simulink model "vtol50kg_hil_chuangheng"  (R2024b)
settings: Solver=FixedStepAuto  StartTime=0.0  StopTime=inf  FixedStep=5/1000  RelTol=1e-3
libraries: slrealtimeutilitieslib x42, slrealtimeiplib x3, simulink x2, aerolibatmos2 x1, hdlsllib x1
settings Model: DataDictionary=nextpilot_datadict.sldd  Creator=CETCA  LastModifiedBy=CETCA
settings DataIOCC: ExternalInput=getinputstruct(report8)  InitialState=getstatestruct(report8)

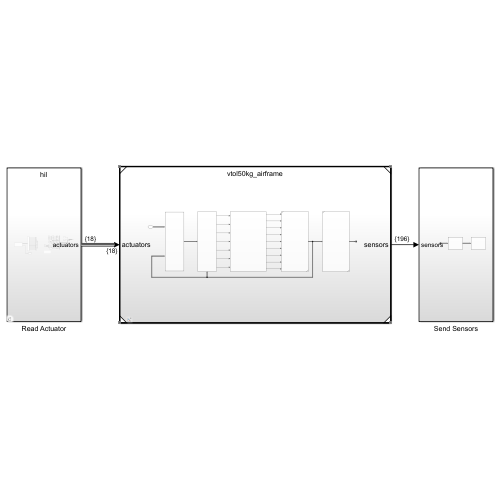
[thumbnail: Simulink's stored preview of the top-level diagram]
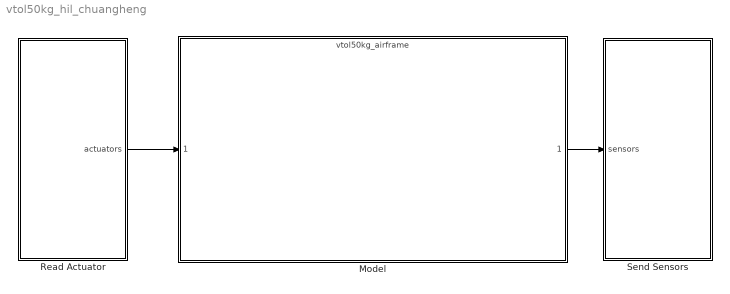
== system vtol50kg_hil_chuangheng ==
  Model : ModelReference  ModelNameDialog=vtol50kg_airframe.slx  SimulationMode=Normal  ModelReferenceVersion=5.134
  Read Actuator : Subsystem  Variant=on
  Send Sensors : Subsystem
  wires:
  Read Actuator/1(actuators) -> Model/1
  Model/1 -> Send Sensors/1(sensors)

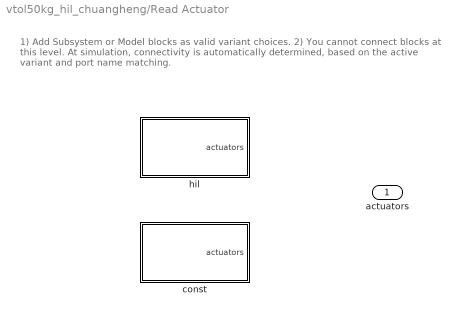
== system vtol50kg_hil_chuangheng/Read Actuator ==
  note: 1) Add Subsystem or Model blocks as valid variant choices.
      | 2) You cannot connect blocks at this level. At simulation, connectivity is automatically
      | determined, based on the active variant and port name matching.
  const : Subsystem  VariantControl=false
  hil : Subsystem  VariantControl=true
  actuators : Outport

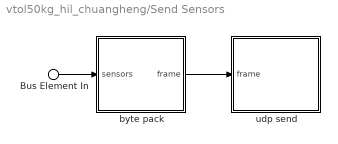
== system vtol50kg_hil_chuangheng/Send Sensors ==
  Bus Element In : Inport  PortName=sensors
  byte pack : Subsystem
  udp send : Subsystem
  wires:
  byte pack/1(frame) -> udp send/1(frame)
  Bus Element In/1 -> byte pack/1(sensors)

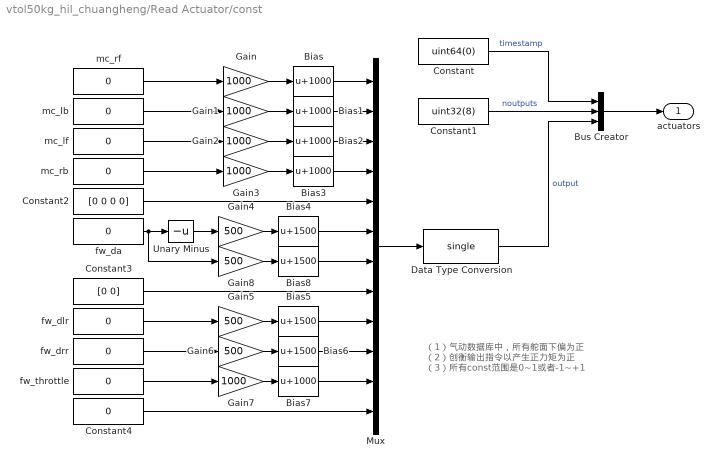
== system vtol50kg_hil_chuangheng/Read Actuator/const ==
  note: （1）气动数据库中，所有舵面下偏为正
      | （2）创衡输出指令以产生正力矩为正
      | （3）所有const范围是0~1或者-1~+1
  Bias{,1..3,7} (5 alike) : Bias  Bias=1000  SaturateOnIntegerOverflow=off
  Bias{4..6,8} (4 alike) : Bias  Bias=1500  SaturateOnIntegerOverflow=off
  Bus Creator : BusCreator  Inputs=3
  Constant : Constant  Value=uint64(0)
  Constant1 : Constant  Value=uint32(8)
  Constant2 : Constant  Value=[0 0 0 0]
  Constant3 : Constant  Value=[0 0]
  Constant4 : Constant  Value=0
  Data Type Conversion : DataTypeConversion  OutDataTypeStr=single  SaturateOnIntegerOverflow=off  RndMeth=Floor
  Gain{,1..3,7} (5 alike) : Gain  Gain=1000
  Gain{4..6,8} (4 alike) : Gain  Gain=500
  Mux : Mux  Inputs=12
  Unary Minus : UnaryMinus
  fw_da : Constant  Value=0
  fw_dlr : Constant  Value=0
  fw_drr : Constant  Value=0
  fw_throttle : Constant  Value=0
  mc_lb : Constant  Value=0
  mc_lf : Constant  Value=0
  mc_rb : Constant  Value=0
  mc_rf : Constant  Value=0
  actuators : Outport
  wires:
  mc_rf/1 -> Gain/1
  fw_dlr/1 -> Gain5/1
  mc_rb/1 -> Gain3/1
  Constant3/1 -> Mux/8
  fw_drr/1 -> Gain6/1
  Data Type Conversion/1 -> Bus Creator/3  "output"
  Gain6/1 -> Bias6/1
  fw_throttle/1 -> Gain7/1
  mc_lb/1 -> Gain1/1
  Bias/1 -> Mux/1
  Mux/1 -> Data Type Conversion/1
  Bus Creator/1 -> actuators/1
  Gain2/1 -> Bias2/1
  Constant1/1 -> Bus Creator/2  "noutputs"
  Gain1/1 -> Bias1/1
  Gain8/1 -> Bias8/1
  Bias2/1 -> Mux/3
  Bias1/1 -> Mux/2
  Bias4/1 -> Mux/6
  Gain7/1 -> Bias7/1
  Gain4/1 -> Bias4/1
  fw_da/1 -> Gain8/1, Unary Minus/1
  Gain/1 -> Bias/1
  Constant4/1 -> Mux/12
  Gain3/1 -> Bias3/1
  Bias5/1 -> Mux/9
  Bias6/1 -> Mux/10
  mc_lf/1 -> Gain2/1
  Bias8/1 -> Mux/7
  Constant/1 -> Bus Creator/1  "timestamp"
  Gain5/1 -> Bias5/1
  Bias3/1 -> Mux/4
  Bias7/1 -> Mux/11
  Constant2/1 -> Mux/5
  Unary Minus/1 -> Gain4/1

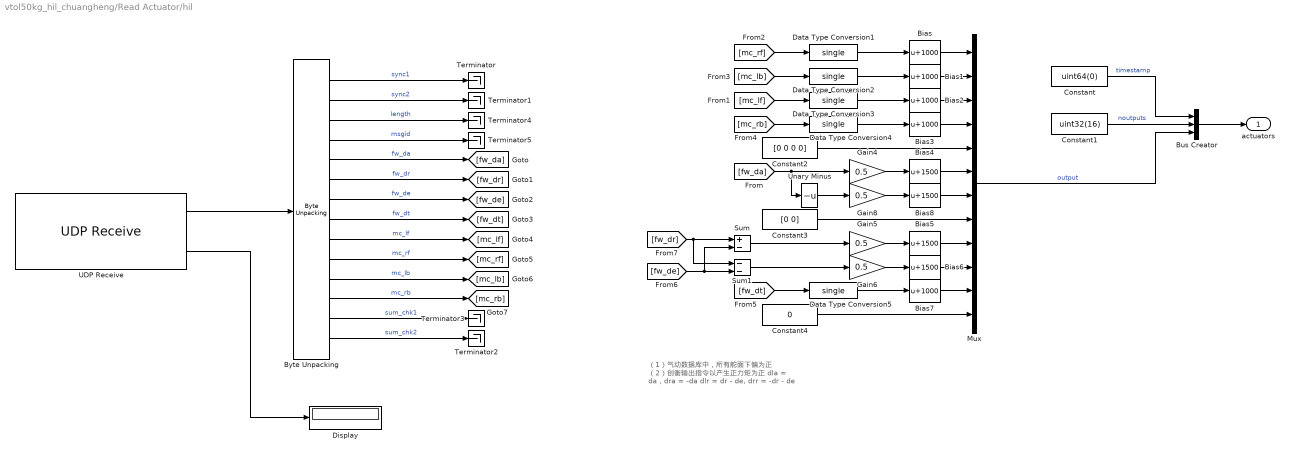
== system vtol50kg_hil_chuangheng/Read Actuator/hil ==
  note: （1）气动数据库中，所有舵面下偏为正
      | （2）创衡输出指令以产生正力矩为正
      |
      | dla = da，dra = -da
      | dlr = dr - de, drr = -dr - de
  Bias{,1..3,7} (5 alike) : Bias  Bias=1000  SaturateOnIntegerOverflow=off
  Bias{4..6,8} (4 alike) : Bias  Bias=1500  SaturateOnIntegerOverflow=off
  Bus Creator : BusCreator  Inputs=3
  Byte Unpacking : slrealtimeutilitieslib/Byte Unpacking  MaskUnpackedDataTypes={'uint8','uint8','uint8','uint8','int16','int16','int16','int16','int16','int16','int16','int16','uint8','uint8'}  MaskUnpackedDataSizes={1,1,1,1,1,1,1,1,1,1,1,1,1,1}  MaskAlignment=1
  Constant : Constant  Value=uint64(0)
  Constant1 : Constant  Value=uint32(16)
  Constant2 : Constant  Value=[0 0 0 0]  OutDataTypeStr=single
  Constant3 : Constant  Value=[0 0]  OutDataTypeStr=single
  Constant4 : Constant  Value=0  OutDataTypeStr=single
  Data Type Conversion{1..5} (5 alike) : DataTypeConversion  OutDataTypeStr=single  SaturateOnIntegerOverflow=off  RndMeth=Floor
  Display : Display
  Gain{4..6,8} (4 alike) : Gain  Gain=0.5  OutDataTypeStr=single
  Mux : Mux  Inputs=12
  Sum : Sum  Inputs=+-
  Sum1 : Sum  Inputs=--
  Terminator{,1..5} (6 alike) : Terminator
  UDP Receive : slrealtimeiplib/UDP Receive  useHostTargetConn=off  ipAddress=192.168.101.56  localPort=8011  rcvWidth=22  rcvFmAny=on  fmAddress='10.10.10.10'  sampleTime=0.01  enableMessage=off  maxPackets=1
  Unary Minus : UnaryMinus
  actuators : Outport
  wires:
  Sum/1 -> Gain5/1
  Constant3/1 -> Mux/8
  Unary Minus/1 -> Gain8/1
  Sum1/1 -> Gain6/1
  Mux/1 -> Bus Creator/3  "output"
  Gain6/1 -> Bias6/1
  Bias/1 -> Mux/1
  Bus Creator/1 -> actuators/1
  [mc_lf] -> Data Type Conversion3/1
  Constant1/1 -> Bus Creator/2  "noutputs"
  [mc_lb] -> Data Type Conversion2/1
  Gain8/1 -> Bias8/1
  Bias2/1 -> Mux/3
  Bias1/1 -> Mux/2
  Bias4/1 -> Mux/6
  [fw_dt] -> Data Type Conversion5/1
  Gain4/1 -> Bias4/1
  [fw_da] -> Unary Minus/1, Gain4/1
  [mc_rf] -> Data Type Conversion1/1
  Constant4/1 -> Mux/12
  [mc_rb] -> Data Type Conversion4/1
  Bias5/1 -> Mux/9
  Bias6/1 -> Mux/10
  Bias8/1 -> Mux/7
  Constant/1 -> Bus Creator/1  "timestamp"
  Gain5/1 -> Bias5/1
  Bias3/1 -> Mux/4
  Bias7/1 -> Mux/11
  Constant2/1 -> Mux/5
  Byte Unpacking/13 -> Terminator3/1  "sum_chk1"
  Byte Unpacking/6 -> [fw_dr]  "fw_dr"
  Byte Unpacking/3 -> Terminator4/1  "length"
  Byte Unpacking/2 -> Terminator1/1  "sync2"
  Byte Unpacking/1 -> Terminator/1  "sync1"
  Byte Unpacking/4 -> Terminator5/1  "msgid"
  UDP Receive/2 -> Display/1
  Byte Unpacking/12 -> [mc_rb]  "mc_rb"
  UDP Receive/1 -> Byte Unpacking/1
  Byte Unpacking/5 -> [fw_da]  "fw_da"
  Byte Unpacking/7 -> [fw_de]  "fw_de"
  Byte Unpacking/14 -> Terminator2/1  "sum_chk2"
  Byte Unpacking/10 -> [mc_rf]  "mc_rf"
  Byte Unpacking/8 -> [fw_dt]  "fw_dt"
  Byte Unpacking/9 -> [mc_lf]  "mc_lf"
  Byte Unpacking/11 -> [mc_lb]  "mc_lb"
  [fw_de] -> Sum/2, Sum1/2
  [fw_dr] -> Sum1/1, Sum/1
  Data Type Conversion1/1 -> Bias/1
  Data Type Conversion2/1 -> Bias1/1
  Data Type Conversion3/1 -> Bias2/1
  Data Type Conversion4/1 -> Bias3/1
  Data Type Conversion5/1 -> Bias7/1

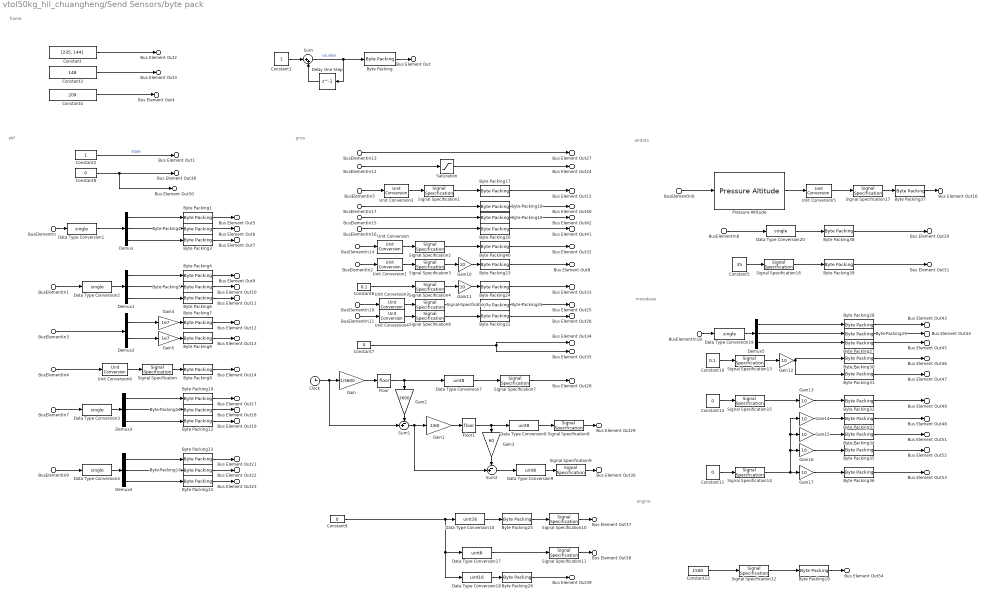
== system vtol50kg_hil_chuangheng/Send Sensors/byte pack ==
  note: frame
  note: engine
  note: movebase
  note: airdata
  note: gnss
  note: ekf
  BusElementIn : Inport  PortName=sensors  Element=states.aircraft.attitude.phi_theta_psi
  BusElementIn1 : Inport  PortName=sensors  Element=states.aircraft.attitude.p_q_r
  BusElementIn3 : Inport  PortName=sensors  Element=states.aircraft.position.lat_lon
  BusElementIn4 : Inport  PortName=sensors  Element=states.aircraft.position.alt
  BusElementIn7 : Inport  PortName=sensors  Element=states.aircraft.position.vn_ve_vd
  BusElementIn9 : Inport  PortName=sensors  Element=states.aircraft.position.an_ae_ad
  BusElementIn18 : Inport  PortName=sensors  Element=states.aircraft.position.pn_pe_pd
  BusElementIn8 : Inport  PortName=sensors  Element=states.aircraft.airdata.airspeed
  BusElementIn2 : Inport  PortName=sensors  Element=gps.heading
  BusElementIn5 : Inport  PortName=sensors  Element=gps.alt
  BusElementIn10 : Inport  PortName=sensors  Element=gps.hdop
  BusElementIn11 : Inport  PortName=sensors  Element=gps.vdop
  BusElementIn12 : Inport  PortName=sensors  Element=gps.satellites_used
  BusElementIn13 : Inport  PortName=sensors  Element=gps.fix_type
  BusElementIn14 : Inport  PortName=sensors  Element=gps.cog_rad
  BusElementIn15 : Inport  PortName=sensors  Element=gps.vel_e_m_s
  BusElementIn16 : Inport  PortName=sensors  Element=gps.vel_d_m_s
  BusElementIn17 : Inport  PortName=sensors  Element=gps.vel_n_m_s
  BusElementIn6 : Inport  PortName=sensors  Element=baro.pressure
  Byte Packing{,1..40} (41 alike) : slrealtimeutilitieslib/Byte Packing
  Clock : Clock
  Constant : Constant  Value=[235, 144]  OutDataTypeStr=uint8
  Constant1 : Constant  OutDataTypeStr=uint32
  Constant10 : Constant  Value=0.1
  Constant11 : Constant  Value=0  OutDataTypeStr=single
  Constant12 : Constant  Value=1500  OutDataTypeStr=uint16
  Constant13 : Constant  Value=0  OutDataTypeStr=single
  Constant2 : Constant  OutDataTypeStr=uint8
  Constant3 : Constant  Value=148  OutDataTypeStr=uint8
  Constant4 : Constant  Value=209  OutDataTypeStr=uint8
  Constant5 : Constant  Value=35  OutDataTypeStr=int8
  Constant6 : Constant  Value=0.1
  Constant7 : Constant  Value=0  OutDataTypeStr=uint8
  Constant8 : Constant  Value=0  OutDataTypeStr=uint8
  Constant9 : Constant  Value=0
  Data Type Conversion{1..4,19..20} (6 alike) : DataTypeConversion  OutDataTypeStr=single  SaturateOnIntegerOverflow=off  RndMeth=Floor
  Data Type Conversion10 : DataTypeConversion  OutDataTypeStr=uint16  SaturateOnIntegerOverflow=off  RndMeth=Floor
  Data Type Conversion{7..9,17} (4 alike) : DataTypeConversion  OutDataTypeStr=uint8  SaturateOnIntegerOverflow=off  RndMeth=Floor
  Data Type Conversion18 : DataTypeConversion  OutDataTypeStr=uint16  SaturateOnIntegerOverflow=off  RndMeth=Floor
  Delay One Step : Delay  DelayLength=1
  Demux{,1,3..5} (5 alike) : Demux  Outputs=3
  Demux2 : Demux  Outputs=2
  Floor : Rounding
  Floor1 : Rounding
  Gain : Gain  Gain=1/3600
  Gain1 : Gain  Gain=1/60
  Gain{10..11,15..17} (5 alike) : Gain  Gain=10  OutDataTypeStr=int16
  Gain12 : Gain  Gain=10  OutDataTypeStr=uint16
  Gain13 : Gain  Gain=10  OutDataTypeStr=uint16
  Gain14 : Gain  Gain=10  OutDataTypeStr=uint16
  Gain2 : Gain  Gain=3600
  Gain3 : Gain  Gain=60
  Gain4 : Gain  Gain=1e7  OutDataTypeStr=int32
  Gain5 : Gain  Gain=1e7  OutDataTypeStr=int32
  Pressure Altitude : aerolibatmos2/Pressure Altitude  units=Metric (MKS)  action=Warning
  Saturation : Saturate  UpperLimit=15  LowerLimit=0
  Signal Specification{,1,5..6,17} (5 alike) : SignalSpecification  Unit=cm
  Signal Specification10 : SignalSpecification  Unit=ms
  Signal Specification11 : SignalSpecification  Unit=d
  Signal Specification12 : SignalSpecification  Unit=rpm
  Signal Specification13 : SignalSpecification  Unit=m
  Signal Specification{2..4,14} (4 alike) : SignalSpecification  Unit=deg
  Signal Specification15 : SignalSpecification  Unit=m/s
  Signal Specification16 : SignalSpecification  Unit=°C
  Signal Specification7 : SignalSpecification  Unit=h
  Signal Specification8 : SignalSpecification  Unit=min
  Signal Specification9 : SignalSpecification  Unit=s
  Sum : Sum  Inputs=|++
  Sum1 : Sum  Inputs=-+|
  Sum2 : Sum  Inputs=-+|
  Unit Conversion : UnitConversion
  Unit Conversion1 : UnitConversion
  Unit Conversion{2..6} (5 alike) : UnitConversion  OutputType=Inherit: Inherit via back propagation
  Bus Element Out2 : Outport  PortName=frame  Element=sync
  Bus Element Out3 : Outport  PortName=frame  Element=length
  Bus Element Out : Outport  PortName=frame  Element=counter
  Bus Element Out4 : Outport  PortName=frame  Element=msgid
  Bus Element Out1 : Outport  PortName=frame  Element=sensor_state
  Bus Element Out6 : Outport  PortName=frame  Element=pitch
  Bus Element Out5 : Outport  PortName=frame  Element=roll
  Bus Element Out7 : Outport  PortName=frame  Element=yaw
  Bus Element Out32 : Outport  PortName=frame  Element=gps_cog
  Bus Element Out10 : Outport  PortName=frame  Element=pitch_rate
  Bus Element Out9 : Outport  PortName=frame  Element=roll_rate
  Bus Element Out11 : Outport  PortName=frame  Element=yaw_rate
  Bus Element Out12 : Outport  PortName=frame  Element=lat
  Bus Element Out13 : Outport  PortName=frame  Element=lon
  Bus Element Out16 : Outport  PortName=frame  Element=baro_alt
  Bus Element Out15 : Outport  PortName=frame  Element=gps_alt
  Bus Element Out14 : Outport  PortName=frame  Element=alt
  Bus Element Out17 : Outport  PortName=frame  Element=vel_n
  Bus Element Out18 : Outport  PortName=frame  Element=vel_e
  Bus Element Out19 : Outport  PortName=frame  Element=vel_d
  Bus Element Out20 : Outport  PortName=frame  Element=airspd
  Bus Element Out21 : Outport  PortName=frame  Element=acc_n
  Bus Element Out22 : Outport  PortName=frame  Element=acc_e
  Bus Element Out23 : Outport  PortName=frame  Element=acc_d
  Bus Element Out24 : Outport  PortName=frame  Element=gps_satellites_used
  Bus Element Out25 : Outport  PortName=frame  Element=gps_hdop
  Bus Element Out26 : Outport  PortName=frame  Element=gps_vdop
  Bus Element Out27 : Outport  PortName=frame  Element=gps_status
  Bus Element Out28 : Outport  PortName=frame  Element=gps_hour
  Bus Element Out29 : Outport  PortName=frame  Element=gps_minute
  Bus Element Out30 : Outport  PortName=frame  Element=gps_second
  Bus Element Out31 : Outport  PortName=frame  Element=imu_temp
  Bus Element Out8 : Outport  PortName=frame  Element=gps_hdg
  Bus Element Out33 : Outport  PortName=frame  Element=gps_hdg_dev
  Bus Element Out50 : Outport  PortName=frame  Element=redundancy
  Bus Element Out34 : Outport  PortName=frame  Element=gps_0_dt
  Bus Element Out35 : Outport  PortName=frame  Element=gps_1_dt
  Bus Element Out36 : Outport  PortName=frame  Element=ahrs_state
  Bus Element Out40 : Outport  PortName=frame  Element=gps_vn
  Bus Element Out42 : Outport  PortName=frame  Element=gps_ve
  Bus Element Out41 : Outport  PortName=frame  Element=gps_vd
  Bus Element Out37 : Outport  PortName=frame  Element=gps_week_ms
  Bus Element Out38 : Outport  PortName=frame  Element=gps_week_day
  Bus Element Out39 : Outport  PortName=frame  Element=gps_week
  Bus Element Out43 : Outport  PortName=frame  Element=align_north
  Bus Element Out44 : Outport  PortName=frame  Element=align_east
  Bus Element Out45 : Outport  PortName=frame  Element=align_up
  Bus Element Out46 : Outport  PortName=frame  Element=align_hpos_std
  Bus Element Out47 : Outport  PortName=frame  Element=align_vpos_std
  Bus Element Out48 : Outport  PortName=frame  Element=boat_cog
  Bus Element Out49 : Outport  PortName=frame  Element=boat_spd
  Bus Element Out54 : Outport  PortName=frame  Element=engine_rpm
  Bus Element Out51 : Outport  PortName=frame  Element=boat_pitch
  Bus Element Out52 : Outport  PortName=frame  Element=boat_roll
  Bus Element Out53 : Outport  PortName=frame  Element=boat_yaw
  wires:
  Constant1/1 -> Sum/1
  Sum/1 -> Delay One Step/1, Byte Packing/1  "counter"
  Delay One Step/1 -> Sum/2
  Constant2/1 -> Bus Element Out1/1  "state"
  BusElementIn/1 -> Data Type Conversion1/1
  Constant/1 -> Bus Element Out2/1
  Constant3/1 -> Bus Element Out3/1
  Constant4/1 -> Bus Element Out4/1
  BusElementIn2/1 -> Unit Conversion1/1
  BusElementIn1/1 -> Data Type Conversion2/1
  BusElementIn3/1 -> Demux2/1
  Demux2/1 -> Gain4/1
  Demux2/2 -> Gain5/1
  BusElementIn6/1 -> Pressure Altitude/1
  BusElementIn7/1 -> Data Type Conversion3/1
  BusElementIn9/1 -> Data Type Conversion4/1
  BusElementIn12/1 -> Saturation/1
  BusElementIn10/1 -> Unit Conversion3/1
  BusElementIn11/1 -> Unit Conversion4/1
  BusElementIn13/1 -> Bus Element Out27/1
  Floor/1 -> Data Type Conversion7/1, Gain2/1
  Clock/1 -> Sum1/2, Gain/1
  Gain/1 -> Floor/1
  Gain1/1 -> Floor1/1
  Floor1/1 -> Data Type Conversion8/1, Gain3/1
  Sum1/1 -> Sum2/2, Gain1/1
  Gain2/1 -> Sum1/1
  Gain3/1 -> Sum2/1
  Sum2/1 -> Data Type Conversion9/1
  Data Type Conversion7/1 -> Signal Specification7/1
  Data Type Conversion8/1 -> Signal Specification8/1
  Data Type Conversion9/1 -> Signal Specification9/1
  Constant5/1 -> Signal Specification16/1
  Constant6/1 -> Signal Specification4/1
  Constant7/1 -> Bus Element Out35/1, Bus Element Out34/1
  Constant8/1 -> Bus Element Out50/1, Bus Element Out36/1
  Constant9/1 -> Data Type Conversion10/1, Data Type Conversion17/1, Data Type Conversion18/1
  BusElementIn18/1 -> Data Type Conversion19/1
  Demux5/2 -> Byte Packing29/1
  Demux5/3 -> Byte Packing27/1
  Constant10/1 -> Signal Specification13/1
  Constant11/1 -> Signal Specification14/1
  Constant12/1 -> Signal Specification12/1
  Byte Packing/1 -> Bus Element Out/1
  Byte Packing1/1 -> Bus Element Out5/1
  Byte Packing2/1 -> Bus Element Out6/1
  Byte Packing3/1 -> Bus Element Out7/1
  Byte Packing4/1 -> Bus Element Out9/1
  Byte Packing5/1 -> Bus Element Out10/1
  Byte Packing6/1 -> Bus Element Out11/1
  Gain4/1 -> Byte Packing7/1
  Gain5/1 -> Byte Packing8/1
  Byte Packing7/1 -> Bus Element Out12/1
  Byte Packing8/1 -> Bus Element Out13/1
  Byte Packing9/1 -> Bus Element Out14/1
  Byte Packing10/1 -> Bus Element Out17/1
  Byte Packing11/1 -> Bus Element Out18/1
  Byte Packing12/1 -> Bus Element Out19/1
  Byte Packing13/1 -> Bus Element Out21/1
  Byte Packing14/1 -> Bus Element Out22/1
  Byte Packing15/1 -> Bus Element Out23/1
  Byte Packing16/1 -> Bus Element Out54/1
  Byte Packing17/1 -> Bus Element Out15/1
  Byte Packing18/1 -> Bus Element Out40/1
  Byte Packing19/1 -> Bus Element Out42/1
  Byte Packing20/1 -> Bus Element Out41/1
  Signal Specification5/1 -> Byte Packing21/1
  Signal Specification6/1 -> Byte Packing22/1
  Byte Packing21/1 -> Bus Element Out25/1
  Byte Packing22/1 -> Bus Element Out26/1
  BusElementIn14/1 -> Unit Conversion/1
  Gain10/1 -> Byte Packing23/1
  Byte Packing23/1 -> Bus Element Out8/1
  Gain11/1 -> Byte Packing24/1
  Byte Packing24/1 -> Bus Element Out33/1
  Data Type Conversion10/1 -> Byte Packing25/1
  Byte Packing25/1 -> Signal Specification10/1
  Data Type Conversion17/1 -> Signal Specification11/1
  Data Type Conversion18/1 -> Byte Packing26/1
  Byte Packing26/1 -> Bus Element Out39/1
  Demux5/1 -> Byte Packing28/1
  Byte Packing27/1 -> Bus Element Out45/1
  Byte Packing28/1 -> Bus Element Out43/1
  Data Type Conversion19/1 -> Demux5/1
  Byte Packing29/1 -> Bus Element Out44/1
  Byte Packing30/1 -> Bus Element Out46/1
  Byte Packing31/1 -> Bus Element Out47/1
  Gain12/1 -> Byte Packing31/1, Byte Packing30/1
  Gain13/1 -> Byte Packing32/1
  Gain14/1 -> Byte Packing33/1
  Byte Packing32/1 -> Bus Element Out49/1
  Byte Packing33/1 -> Bus Element Out48/1
  Gain15/1 -> Byte Packing34/1
  Gain16/1 -> Byte Packing35/1
  Byte Packing34/1 -> Bus Element Out51/1
  Byte Packing35/1 -> Bus Element Out52/1
  Gain17/1 -> Byte Packing36/1
  Byte Packing36/1 -> Bus Element Out53/1
  Signal Specification17/1 -> Byte Packing37/1
  Byte Packing37/1 -> Bus Element Out16/1
  Data Type Conversion20/1 -> Byte Packing38/1
  Byte Packing38/1 -> Bus Element Out20/1
  Demux/1 -> Byte Packing1/1
  Demux/2 -> Byte Packing2/1
  Demux/3 -> Byte Packing3/1
  Demux1/1 -> Byte Packing4/1
  Demux1/2 -> Byte Packing5/1
  Demux1/3 -> Byte Packing6/1
  Demux4/1 -> Byte Packing13/1
  Demux4/2 -> Byte Packing14/1
  Demux4/3 -> Byte Packing15/1
  Demux3/1 -> Byte Packing10/1
  Demux3/2 -> Byte Packing11/1
  Demux3/3 -> Byte Packing12/1
  Signal Specification/1 -> Byte Packing9/1
  Signal Specification1/1 -> Byte Packing17/1
  Unit Conversion/1 -> Signal Specification2/1
  Unit Conversion1/1 -> Signal Specification3/1
  Signal Specification4/1 -> Gain11/1
  Unit Conversion3/1 -> Signal Specification5/1
  Unit Conversion4/1 -> Signal Specification6/1
  Signal Specification7/1 -> Bus Element Out28/1
  Signal Specification8/1 -> Bus Element Out29/1
  Signal Specification9/1 -> Bus Element Out30/1
  Signal Specification10/1 -> Bus Element Out37/1
  Signal Specification11/1 -> Bus Element Out38/1
  Signal Specification12/1 -> Byte Packing16/1
  Signal Specification13/1 -> Gain12/1
  Signal Specification14/1 -> Gain14/1, Gain15/1, Gain16/1, Gain17/1
  Constant13/1 -> Signal Specification15/1
  Signal Specification15/1 -> Gain13/1
  Signal Specification16/1 -> Byte Packing39/1
  Byte Packing39/1 -> Bus Element Out31/1
  Byte Packing40/1 -> Bus Element Out32/1
  Saturation/1 -> Bus Element Out24/1
  Pressure Altitude/1 -> Unit Conversion5/1
  BusElementIn5/1 -> Unit Conversion2/1
  BusElementIn4/1 -> Unit Conversion6/1
  Unit Conversion5/1 -> Signal Specification17/1
  BusElementIn8/1 -> Data Type Conversion20/1
  BusElementIn17/1 -> Byte Packing18/1
  BusElementIn15/1 -> Byte Packing19/1
  BusElementIn16/1 -> Byte Packing20/1
  Signal Specification2/1 -> Byte Packing40/1
  Signal Specification3/1 -> Gain10/1
  Unit Conversion2/1 -> Signal Specification1/1
  Data Type Conversion1/1 -> Demux/1
  Data Type Conversion2/1 -> Demux1/1
  Unit Conversion6/1 -> Signal Specification/1
  Data Type Conversion3/1 -> Demux3/1
  Data Type Conversion4/1 -> Demux4/1

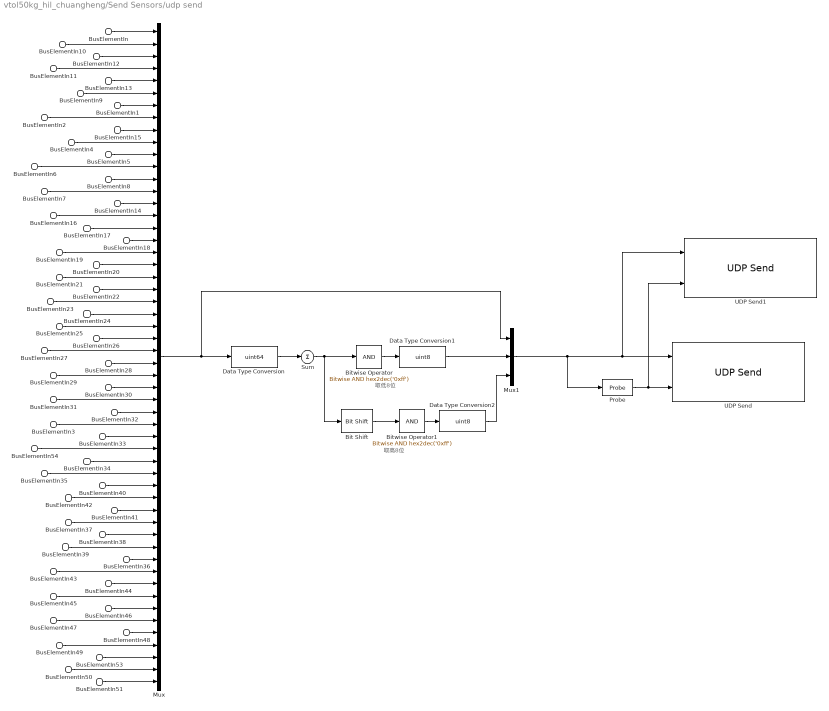
== system vtol50kg_hil_chuangheng/Send Sensors/udp send ==
  note: 取低8位
  note: 取高8位
  BusElementIn : Inport  PortName=frame  Element=sync
  BusElementIn1 : Inport  PortName=frame  Element=roll
  BusElementIn2 : Inport  PortName=frame  Element=yaw
  BusElementIn3 : Inport  PortName=frame  Element=gps_hdg
  BusElementIn4 : Inport  PortName=frame  Element=pitch_rate
  BusElementIn5 : Inport  PortName=frame  Element=roll_rate
  BusElementIn6 : Inport  PortName=frame  Element=yaw_rate
  BusElementIn7 : Inport  PortName=frame  Element=lat
  BusElementIn8 : Inport  PortName=frame  Element=lon
  BusElementIn9 : Inport  PortName=frame  Element=pitch
  BusElementIn10 : Inport  PortName=frame  Element=length
  BusElementIn11 : Inport  PortName=frame  Element=counter
  BusElementIn12 : Inport  PortName=frame  Element=msgid
  BusElementIn13 : Inport  PortName=frame  Element=sensor_state
  BusElementIn15 : Inport  PortName=frame  Element=gps_cog
  BusElementIn14 : Inport  PortName=frame  Element=baro_alt
  BusElementIn16 : Inport  PortName=frame  Element=gps_alt
  BusElementIn17 : Inport  PortName=frame  Element=alt
  BusElementIn18 : Inport  PortName=frame  Element=vel_n
  BusElementIn19 : Inport  PortName=frame  Element=vel_e
  BusElementIn20 : Inport  PortName=frame  Element=vel_d
  BusElementIn21 : Inport  PortName=frame  Element=airspd
  BusElementIn22 : Inport  PortName=frame  Element=acc_n
  BusElementIn23 : Inport  PortName=frame  Element=acc_e
  BusElementIn24 : Inport  PortName=frame  Element=acc_d
  BusElementIn25 : Inport  PortName=frame  Element=gps_satellites_used
  BusElementIn26 : Inport  PortName=frame  Element=gps_hdop
  BusElementIn27 : Inport  PortName=frame  Element=gps_vdop
  BusElementIn28 : Inport  PortName=frame  Element=gps_status
  BusElementIn29 : Inport  PortName=frame  Element=gps_hour
  BusElementIn30 : Inport  PortName=frame  Element=gps_minute
  BusElementIn31 : Inport  PortName=frame  Element=gps_second
  BusElementIn32 : Inport  PortName=frame  Element=imu_temp
  BusElementIn33 : Inport  PortName=frame  Element=gps_hdg_dev
  BusElementIn34 : Inport  PortName=frame  Element=gps_0_dt
  BusElementIn35 : Inport  PortName=frame  Element=gps_1_dt
  BusElementIn36 : Inport  PortName=frame  Element=ahrs_state
  BusElementIn37 : Inport  PortName=frame  Element=gps_week_ms
  BusElementIn38 : Inport  PortName=frame  Element=gps_week_day
  BusElementIn39 : Inport  PortName=frame  Element=gps_week
  BusElementIn40 : Inport  PortName=frame  Element=gps_vn
  BusElementIn41 : Inport  PortName=frame  Element=gps_vd
  BusElementIn42 : Inport  PortName=frame  Element=gps_ve
  BusElementIn43 : Inport  PortName=frame  Element=align_north
  BusElementIn44 : Inport  PortName=frame  Element=align_east
  BusElementIn45 : Inport  PortName=frame  Element=align_up
  BusElementIn46 : Inport  PortName=frame  Element=align_hpos_std
  BusElementIn47 : Inport  PortName=frame  Element=align_vpos_std
  BusElementIn48 : Inport  PortName=frame  Element=boat_cog
  BusElementIn49 : Inport  PortName=frame  Element=boat_spd
  BusElementIn50 : Inport  PortName=frame  Element=boat_pitch
  BusElementIn51 : Inport  PortName=frame  Element=boat_roll
  BusElementIn53 : Inport  PortName=frame  Element=engine_rpm
  BusElementIn54 : Inport  PortName=frame  Element=redundancy
  Bit Shift : hdlsllib/Logic and Bit Operations/Bit Shift  mode=Shift Right Logical  N=8
  Bitwise Operator : simulink/Logic and Bit Operations/Bitwise Operator  logicop=AND  UseBitMask=on  BitMask=hex2dec('0xff')  BitMaskRealWorld=Stored Integer
  Bitwise Operator1 : simulink/Logic and Bit Operations/Bitwise Operator  logicop=AND  UseBitMask=on  BitMask=hex2dec('0xff')  BitMaskRealWorld=Stored Integer
  Data Type Conversion : DataTypeConversion  OutDataTypeStr=uint64  SaturateOnIntegerOverflow=off  RndMeth=Floor
  Data Type Conversion1 : DataTypeConversion  OutDataTypeStr=uint8  SaturateOnIntegerOverflow=off  RndMeth=Floor
  Data Type Conversion2 : DataTypeConversion  OutDataTypeStr=uint8  SaturateOnIntegerOverflow=off  RndMeth=Floor
  Mux : Mux  Inputs=54
  Mux1 : Mux  Inputs=3
  Probe : Probe  ProbeSampleTime=off  ProbeComplexSignal=off
  Sum : Sum  Inputs=1
  UDP Send : slrealtimeiplib/UDP Send  useHostTargetConn=off  toAddress='192.168.101.101'  toPort=8012  sampleTime=-1  enableMessage=off
  UDP Send1 : slrealtimeiplib/UDP Send  useHostTargetConn=off  toAddress='192.168.101.20'  toPort=8012  sampleTime=-1  enableMessage=off
  wires:
  BusElementIn/1 -> Mux/1
  BusElementIn10/1 -> Mux/2
  BusElementIn12/1 -> Mux/3
  BusElementIn11/1 -> Mux/4
  BusElementIn13/1 -> Mux/5
  BusElementIn9/1 -> Mux/6
  BusElementIn1/1 -> Mux/7
  BusElementIn2/1 -> Mux/8
  BusElementIn15/1 -> Mux/9
  BusElementIn4/1 -> Mux/10
  BusElementIn5/1 -> Mux/11
  BusElementIn6/1 -> Mux/12
  BusElementIn7/1 -> Mux/14
  BusElementIn8/1 -> Mux/13
  BusElementIn14/1 -> Mux/15
  BusElementIn16/1 -> Mux/16
  BusElementIn17/1 -> Mux/17
  BusElementIn18/1 -> Mux/18
  BusElementIn19/1 -> Mux/19
  BusElementIn20/1 -> Mux/20
  BusElementIn21/1 -> Mux/21
  BusElementIn22/1 -> Mux/22
  BusElementIn23/1 -> Mux/23
  BusElementIn24/1 -> Mux/24
  Mux/1 -> Mux1/1, Data Type Conversion/1
  BusElementIn25/1 -> Mux/25
  BusElementIn26/1 -> Mux/26
  BusElementIn27/1 -> Mux/27
  BusElementIn28/1 -> Mux/28
  BusElementIn29/1 -> Mux/29
  BusElementIn30/1 -> Mux/30
  BusElementIn31/1 -> Mux/31
  BusElementIn32/1 -> Mux/32
  BusElementIn3/1 -> Mux/33
  BusElementIn33/1 -> Mux/34
  BusElementIn54/1 -> Mux/35
  BusElementIn34/1 -> Mux/36
  BusElementIn35/1 -> Mux/37
  BusElementIn40/1 -> Mux/38
  BusElementIn42/1 -> Mux/39
  BusElementIn41/1 -> Mux/40
  BusElementIn37/1 -> Mux/41
  BusElementIn38/1 -> Mux/42
  BusElementIn39/1 -> Mux/43
  BusElementIn36/1 -> Mux/44
  BusElementIn43/1 -> Mux/45
  BusElementIn44/1 -> Mux/46
  BusElementIn45/1 -> Mux/47
  BusElementIn46/1 -> Mux/48
  BusElementIn47/1 -> Mux/49
  BusElementIn48/1 -> Mux/50
  BusElementIn49/1 -> Mux/51
  BusElementIn53/1 -> Mux/52
  BusElementIn50/1 -> Mux/53
  BusElementIn51/1 -> Mux/54
  Data Type Conversion/1 -> Sum/1
  Sum/1 -> Bit Shift/1, Bitwise Operator/1
  Bit Shift/1 -> Bitwise Operator1/1
  Bitwise Operator/1 -> Data Type Conversion1/1
  Bitwise Operator1/1 -> Data Type Conversion2/1
  Data Type Conversion1/1 -> Mux1/2
  Data Type Conversion2/1 -> Mux1/3
  Mux1/1 -> Probe/1, UDP Send1/1, UDP Send/1
  Probe/1 -> UDP Send1/2, UDP Send/2
